simulink model "LLC_Reverse"  (R2024a)
settings: Solver=FixedStepDiscrete  StartTime=0.0  StopTime=0.3  FixedStep=Ts_Power  RelTol=1e-3  EnableMultiTasking=on
values from neighbouring files (symbols this model uses):
  Co = 560e-6    (= 0.00056)    [LLC_Data.m]    (also in LLC_Reverse_Data.m)
  Cr = 140e-9    (= 1.4e-07)    [LLC_Data.m]    (also in LLC_Reverse_Data.m)
  fs_LCC_max = 250e3    (= 250000)    [LLC_Data.m]    (also in LLC_Reverse_Data.m)
  fs_LCC_min = 40e3    (= 40000)    [LLC_Data.m]    (also in LLC_Reverse_Data.m)
  Ki_LLC = 500e3    (= 500000)    [LLC_Data.m]    (also in LLC_Reverse_Data.m)
  Kp_LLC = 5e3    (= 5000)    [LLC_Data.m]    (also in LLC_Reverse_Data.m)
  Lm = 100e-6    (= 0.0001)    [LLC_Data.m]    (also in LLC_Reverse_Data.m)
  Lr = 20e-6    (= 2e-05)    [LLC_Data.m]    (also in LLC_Reverse_Data.m)
  Np = 11    [LLC_Data.m]    (also in LLC_Reverse_Data.m)
  Ns = 10    [LLC_Data.m]    (also in LLC_Reverse_Data.m)
  Ro = Vo_nom^2/Po_nom    (= 19.6363636364)    [LLC_Data.m]    (also in LLC_Reverse_Data.m)
  Ts_Control = 10e-6    (= 1e-05)    [LLC_Data.m]    (also in LLC_Reverse_Data.m)
  Ts_Power = 50e-9    (= 5e-08)    [LLC_Data.m]    (also in LLC_Reverse_Data.m)
  V_o_max = 450    [LLC_Data.m]    (also in LLC_Reverse_Data.m)
  V_o_min = 275    [LLC_Data.m]    (also in LLC_Reverse_Data.m)
undefined symbols (not defined in the file or in its folder): DiscIntNeverNeededParam
libraries: spsMosfetLib x8, spsVoltageMeasurementLib x5, spsSeriesRLCBranchLib x4, spsOnDelayLib x4, spsCurrentMeasurementLib x3, slpidlib x2, spsControlledVoltageSourceLib x1, spsLinearTransformerLib x1, spspowerguiLib x1
settings Model: SimulationMode=accelerator  Creator=LWYohann  LastModifiedBy=LWYohann

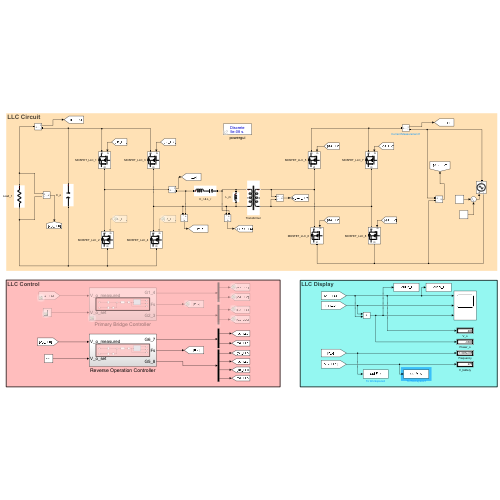
[thumbnail: Simulink's stored preview of the top-level diagram]
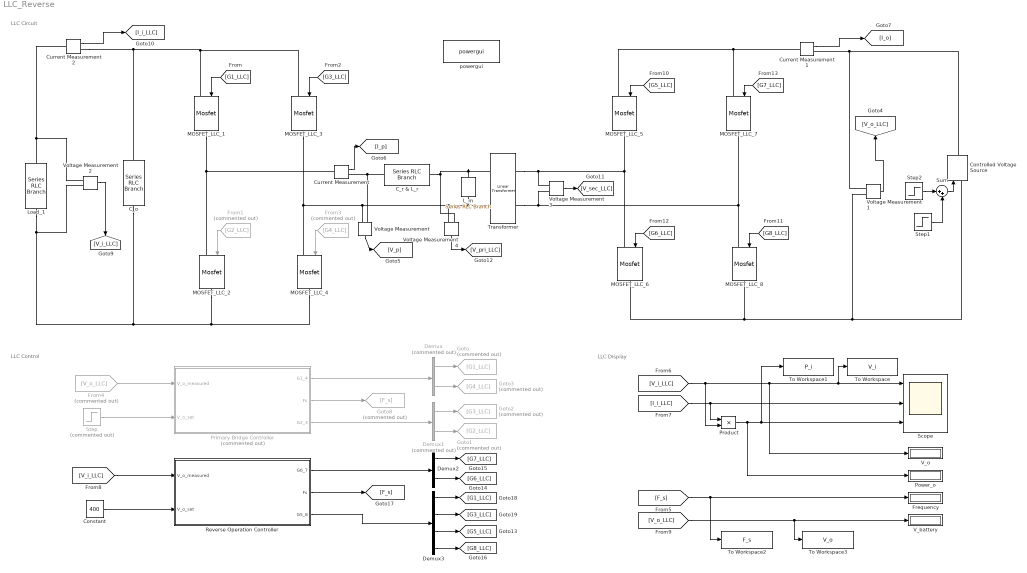
== system LLC_Reverse ==
  note: LLC Display
  note: LLC Control
  note: LLC Circuit
  C_o : spsSeriesRLCBranchLib/Series RLC Branch  LConnTagsString=__new0  RConnTagsString=__new0  BranchType=C  Resistance=1  Inductance=1e-3  SetiL0=off  InitialCurrent=0  Capacitance=Co  Setx0=on  InitialVoltage=400  Measurements=None
  C_r & L_r : spsSeriesRLCBranchLib/Series RLC Branch  LConnTagsString=__new0  RConnTagsString=__new0  BranchType=LC  Resistance=1  Inductance=Lr  SetiL0=off  InitialCurrent=0  Capacitance=Cr  Setx0=off  InitialVoltage=0  Measurements=Branch current
  Constant : Constant  Value=400  SampleTime=Ts_Power
  Controlled Voltage Source : spsControlledVoltageSourceLib/Controlled Voltage Source  Initialize=on  Source_Type=DC  Amplitude=360  Phase=0  Frequency=0  Measurements=None
  Current Measurement : spsCurrentMeasurementLib/Current Measurement  PhasorSimulation=off  OutputType=Complex  PSBequivalent=0
  Current Measurement1 : spsCurrentMeasurementLib/Current Measurement  PhasorSimulation=off  OutputType=Complex  PSBequivalent=0
  Current Measurement2 : spsCurrentMeasurementLib/Current Measurement  PhasorSimulation=off  OutputType=Complex  PSBequivalent=0
  Demux : Demux  Commented=on  Outputs=2
  Demux1 : Demux  Commented=on  Outputs=2
  Demux2 : Demux  Outputs=2
  Demux3 : Demux
  Frequency : Display
  From1 : From  Commented=on  GotoTag=G2_LLC
  From3 : From  Commented=on  GotoTag=G4_LLC
  From4 : From  Commented=on  GotoTag=V_o_LLC
  Goto : Goto  Commented=on  GotoTag=G1_LLC
  Goto1 : Goto  Commented=on  GotoTag=G2_LLC
  Goto2 : Goto  Commented=on  GotoTag=G3_LLC
  Goto3 : Goto  Commented=on  GotoTag=G4_LLC
  Goto8 : Goto  Commented=on  GotoTag=F_s
  L_m : spsSeriesRLCBranchLib/Series RLC Branch  LConnTagsString=__new0  RConnTagsString=__new0  BranchType=L  Resistance=1  Inductance=Lm  SetiL0=off  InitialCurrent=0  Capacitance=Cr  Setx0=off  InitialVoltage=0  Measurements=Branch current
  Load_1 : spsSeriesRLCBranchLib/Series RLC Branch  LConnTagsString=__new0  RConnTagsString=__new0  BranchType=R  Resistance=2*Ro  Inductance=1e-3  SetiL0=off  InitialCurrent=0  Capacitance=Co  Setx0=on  InitialVoltage=375  Measurements=None
  MOSFET_LLC_{1..8} (8 alike) : spsMosfetLib/Mosfet  Ron=Ron_FET  Lon=0  Rd=Ron_Diode  Vfd=Vf  IC=0  Rs=1e6  Cs=inf  Measurements=off
  Power_o : Display
  Primary Bridge Controller : Subsystem  Commented=on
  Product : Product
  Reverse Operation Controller : Subsystem
  Scope : Scope  NumInputPorts=3
  Step : Step  Commented=on  Time=0.1  Before=275  After=360  SampleTime=Ts_Power
  Step1 : Step  Time=0.2  After=-175  SampleTime=Ts_Power
  Step2 : Step  Time=0.1  Before=360  After=450  SampleTime=Ts_Power
  Sum : Sum  Inputs=|++
  To Workspace : ToWorkspace  VariableName=V_i  SaveFormat=Structure With Time  SampleTime=Ts_Power
  To Workspace1 : ToWorkspace  VariableName=P_i  SaveFormat=Structure With Time  SampleTime=Ts_Power
  To Workspace2 : ToWorkspace  VariableName=F_s  SaveFormat=Structure With Time  SampleTime=Ts_Power
  To Workspace3 : ToWorkspace  VariableName=V_o  SaveFormat=Structure With Time  SampleTime=Ts_Power
  Transformer : spsLinearTransformerLib/Linear Transformer  UNITS=SI  NominalPower=[ 6.6e3 100e3 ]  winding1="[Np   1e-2 0]"  winding2="[Ns  1e-2  0 ]"  ThreeWindings=off  winding3=[3.15e+05 0.7938 0.084225]  RmLm=[1e4 0]  Measurements=Magnetization current  DataType=on
  V_battery : Display
  V_o : Display
  Voltage Measurement{,1..4} (5 alike) : spsVoltageMeasurementLib/Voltage Measurement  PhasorSimulation=off  OutputType=Complex  PSBequivalent=0
  powergui : spspowerguiLib/powergui  Priority=1  SimulationMode=Discrete  SampleTime=Ts_Power  frequency=60  Iterations=50  frequencyindice=0  Pbase=100e6  ErrMax=1e-4  UnitsV=kV  UnitsW=MW  buscounter=0  FunctionMessages=off  echomessages=off  EnableUseOfTLC=off  CurrentSourceSwitches=off  DisableSnubberDevices=off  DisableRonSwitches=off  DisableVfSwitches=off  DisplayEquations=off  AutomaticDiscreteSolvers=off  SolverType=Tustin/Backward Euler (TBE)  Interpol=off  ExternalGateDelay=off  methode=off  Ts=100  x0status=blocks  SPID=on  SwTol=0  HookPort=off  NonlinearTolerance=1e-4  nMaxIteration=100  ContinueOnMaxIteration=off  RestoreLinks=warning  ResistiveCurrentMeasurement=off  Frange=[0:2:500]  Ylog=off  Xlog=on  ShowGrid=off  save=off  variable=ZData  structure=0  ZoomFFT=off  StartTime=0.0  cycles=1  DisplayStyle=1  fundamental=60  FreqAxis=off  MaxFrequency=1000  frequencyindicesteady=1  RmsSteady=1  display=off
  wires:
  Demux/1 -> Goto/1
  Demux/2 -> Goto3/1
  Demux1/1 -> Goto2/1
  Demux1/2 -> Goto1/1
  [G1_LLC] -> MOSFET_LLC_1/1
  From1/1 -> MOSFET_LLC_2/1
  [G3_LLC] -> MOSFET_LLC_3/1
  From3/1 -> MOSFET_LLC_4/1
  Voltage Measurement1/1 -> [V_o_LLC]
  Voltage Measurement/1 -> [V_p]
  Current Measurement/1 -> [I_p]
  Current Measurement1/1 -> [I_o]
  [V_i_LLC] -> V_o/1, To Workspace/1, Scope/1, Product/2
  [I_i_LLC] -> Product/1, Scope/2
  Product/1 -> Power_o/1, To Workspace1/1, Scope/3
  [F_s] -> To Workspace2/1, Frequency/1
  Voltage Measurement2/1 -> [V_i_LLC]
  Current Measurement2/1 -> [I_i_LLC]
  Voltage Measurement3/1 -> [V_sec_LLC]
  [G5_LLC] -> MOSFET_LLC_5/1
  [G8_LLC] -> MOSFET_LLC_8/1
  [G6_LLC] -> MOSFET_LLC_6/1
  [G7_LLC] -> MOSFET_LLC_7/1
  Voltage Measurement4/1 -> [V_pri_LLC]
  From4/1 -> Primary Bridge Controller/1(V_o_measured)
  Step/1 -> Primary Bridge Controller/2(V_o_set)
  Primary Bridge Controller/1(G1_4) -> Demux/1
  Primary Bridge Controller/3(G2_3) -> Demux1/1
  Primary Bridge Controller/2(Fs) -> Goto8/1
  [V_i_LLC] -> Reverse Operation Controller/1(V_o_measured)
  Constant/1 -> Reverse Operation Controller/2(V_o_set)
  Reverse Operation Controller/2(Fs) -> [F_s]
  Step2/1 -> Sum/1
  Sum/1 -> Controlled Voltage Source/1
  Step1/1 -> Sum/2
  Reverse Operation Controller/1(G6_7) -> Demux2/1
  Demux2/1 -> [G7_LLC]
  Demux2/2 -> [G6_LLC]
  Reverse Operation Controller/3(G5_8) -> Demux3/1
  Demux3/1 -> [G1_LLC]
  Demux3/2 -> [G3_LLC]
  Demux3/3 -> [G5_LLC]
  Demux3/4 -> [G8_LLC]
  [V_o_LLC] -> To Workspace3/1, V_battery/1
  connections:
  C_r & L_r/RConn1 -- L_m/LConn1 -- Transformer/LConn1 -- Voltage Measurement4/LConn1
  Transformer/LConn2 -- L_m/RConn1 -- Voltage Measurement4/LConn2 -- Voltage Measurement/LConn2 -- MOSFET_LLC_3/RConn1 -- MOSFET_LLC_4/LConn1
  MOSFET_LLC_1/RConn1 -- Current Measurement/LConn1 -- MOSFET_LLC_2/LConn1
  MOSFET_LLC_3/LConn1 -- Current Measurement2/RConn1 -- C_o/LConn1 -- MOSFET_LLC_1/LConn1
  Voltage Measurement2/LConn2 -- Load_1/RConn1 -- C_o/RConn1 -- MOSFET_LLC_4/RConn1 -- MOSFET_LLC_2/RConn1
  Transformer/RConn1 -- Voltage Measurement3/LConn1 -- MOSFET_LLC_6/LConn1 -- MOSFET_LLC_5/RConn1
  Current Measurement1/LConn1 -- MOSFET_LLC_5/LConn1 -- MOSFET_LLC_7/LConn1
  MOSFET_LLC_6/RConn1 -- Voltage Measurement1/LConn2 -- Controlled Voltage Source/LConn1 -- MOSFET_LLC_8/RConn1
  Transformer/RConn2 -- Voltage Measurement3/LConn2 -- MOSFET_LLC_7/RConn1 -- MOSFET_LLC_8/LConn1
  C_r & L_r/LConn1 -- Voltage Measurement/LConn1 -- Current Measurement/RConn1
  Current Measurement2/LConn1 -- Load_1/LConn1 -- Voltage Measurement2/LConn1
  Voltage Measurement1/LConn1 -- Controlled Voltage Source/RConn1 -- Current Measurement1/RConn1

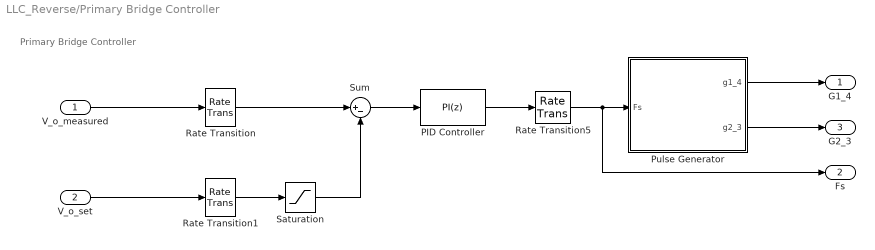
== system LLC_Reverse/Primary Bridge Controller ==
  note: Primary Bridge Controller
  V_o_measured : Inport
  V_o_set : Inport  Port=2
  PID Controller : slpidlib/PID Controller  Controller=PI  Form=Parallel  TimeDomain=Discrete-time  UseExternalTs=off  SampleTime=Ts_Control  IntegratorMethod=Forward Euler  FilterMethod=Forward Euler  ControllerParametersSource=internal  P=Kp_LLC  I=Ki_LLC  UseKiTs=off  D=0  UseExternalDerivativeSource=off  N=100  UseFilter=on  TunerSelectOption=Transfer Function Based (PID Tuner App)  InitialConditionSource=internal  InitialConditionForIntegrator=fr  InitialConditionForFilter=0  DifferentiatorICPrevScaledInput=0  ExternalReset=none  TrackingMode=off  Kt=1  LimitOutput=on  SatLimitsSource=internal  UpperSaturationLimit=fs_LCC_max  LowerSaturationLimit=fs_LCC_min  LinearizeAsGain=on  AntiWindupMode=none  Kb=1  LimitIntegrator=on  UpperIntegratorSaturationLimit=fs_LCC_max  LowerIntegratorSaturationLimit=fs_LCC_min  POutMin=[]  POutMax=[]  IOutMin=[]  IOutMax=[]  DOutMin=[]  DOutMax=[]  NOutMin=[]  NOutMax=[]  SumOutMin=[]  SumOutMax=[]  SaturationOutMin=[]  SaturationOutMax=[]  PParamMin=[]  PParamMax=[]  IParamMin=[]  IParamMax=[]  DParamMin=[]  DParamMax=[]  NParamMin=[]  NParamMax=[]  KbParamMin=[]  KbParamMax=[]  KtParamMin=[]  KtParamMax=[]  KbOutMin=[]  KbOutMax=[]  KtOutMin=[]  KtOutMax=[]  IntegratorOutMin=[]  IntegratorOutMax=[]  FilterOutMin=[]  FilterOutMax=[]  SumI1OutMin=[]  SumI1OutMax=[]  SumI2OutMin=[]  SumI2OutMax=[]  SumI3OutMin=[]  SumI3OutMax=[]  SumI4OutMin=[]  SumI4OutMax=[]  SumDOutMin=[]  SumDOutMax=[]  DifferentiatorOutMin=[]  DifferentiatorOutMax=[]  FilterDiffOutCoefMin=[]  FilterDiffOutCoefMax=[]  ReciprocalOutMin=[]  ReciprocalOutMax=[]  SumDenOutMin=[]  SumDenOutMax=[]  SumNumOutMin=[]  SumNumOutMax=[]  DivideOutMin=[]  DivideOutMax=[]  UdiffTsProdOutMin=[]  UdiffTsProdOutMax=[]  NTsProdOutMin=[]  NTsProdOutMax=[]  UintegralTsProdOutMin=[]  UintegralTsProdOutMax=[]  UngainTsProdOutMin=[]  UngainTsProdOutMax=[]  ClampingZeroOutDataTypeStr=Inherit: Inherit via back propagation  ClampingZeroOutMin=[]  ClampingZeroOutMax=[]  FilterDenConstantOutDataTypeStr=Inherit: Inherit via back propagation  FilterDenConstantOutMin=[]  FilterDenConstantOutMax=[]  PCopyOutDataTypeStr=Inherit: Inherit via back propagation  PCopyOutMin=[]  PCopyOutMax=[]  NCopyOutDataTypeStr=Inherit: Inherit via back propagation  NCopyOutMin=[]  NCopyOutMax=[]  IntegratorContinuousStateAttributes=''  IntegratorStateMustResolveToSignalObject=off  IntegratorRTWStateStorageClass=Auto  FilterContinuousStateAttributes=''  FilterStateMustResolveToSignalObject=off  FilterRTWStateStorageClass=Auto  ParallelPVariant=InternalParameters  IdealPVariant=Disabled  IVariant=InternalParameters  DVariant=Disabled  IntegratorVariant=Discrete  SatVariant=Enabled  AWVariant=Passthrough  PCopyVariant=Disabled  TRVariant=Disabled  FdbkBlocksVariant=Forward  IdealPFdbkVariant=Disabled  SatFdbkVariant=Disabled  DerivativeFilterVariant=Disabled  NVariant=Disabled  NCopyVariant=Disabled_SignalSpec  FilterICVariant=Disabled  IntegratorICVariant=InternalICs  ExternalResetVariant=Disabled  TRSumVariant=Passthrough  SumFdbkVariant=Disabled  SumVariant=Sum_PI  TsampFilterVariant=InternalTs  TsampNgainVariant=Passthrough  TsampIntegralVariant=Disabled_SignalSpec  ExternalSaturationOutDataTypeStr=Inherit: Same as second input  DerivativeSourceVariant=Disabled
  Pulse Generator : Subsystem
  Rate Transition : RateTransition  OutPortSampleTime=Ts_Control
  Rate Transition1 : RateTransition  OutPortSampleTime=Ts_Control
  Rate Transition5 : RateTransition  InitialCondition=fs_LCC_min  OutPortSampleTime=Ts_Power
  Saturation : Saturate  UpperLimit=V_o_max  LowerLimit=V_o_min
  Sum : Sum  Inputs=|+-
  G1_4 : Outport
  Fs : Outport  Port=2
  G2_3 : Outport  Port=3
  wires:
  V_o_measured/1 -> Rate Transition/1
  Pulse Generator/1(g1_4) -> G1_4/1
  Sum/1 -> PID Controller/1
  PID Controller/1 -> Rate Transition5/1
  Rate Transition5/1 -> Fs/1, Pulse Generator/1(Fs)
  Rate Transition/1 -> Sum/1
  V_o_set/1 -> Rate Transition1/1
  Rate Transition1/1 -> Saturation/1
  Saturation/1 -> Sum/2
  Pulse Generator/2(g2_3) -> G2_3/1

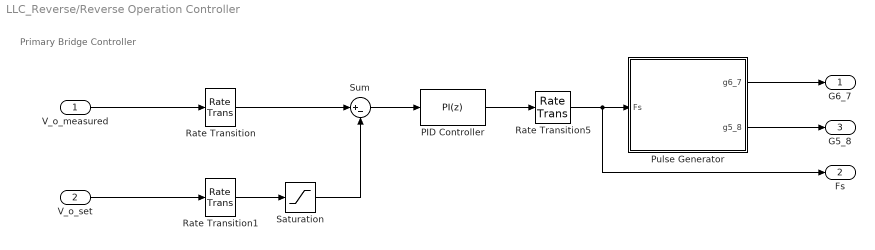
== system LLC_Reverse/Reverse Operation Controller ==
  note: Primary Bridge Controller
  V_o_measured : Inport
  V_o_set : Inport  Port=2
  PID Controller : slpidlib/PID Controller  Controller=PI  Form=Parallel  TimeDomain=Discrete-time  UseExternalTs=off  SampleTime=Ts_Control  IntegratorMethod=Forward Euler  FilterMethod=Forward Euler  ControllerParametersSource=internal  P=Kp_LLC  I=Ki_LLC  UseKiTs=off  D=0  UseExternalDerivativeSource=off  N=100  UseFilter=on  TunerSelectOption=Transfer Function Based (PID Tuner App)  InitialConditionSource=internal  InitialConditionForIntegrator=fr  InitialConditionForFilter=0  DifferentiatorICPrevScaledInput=0  ExternalReset=none  TrackingMode=off  Kt=1  LimitOutput=on  SatLimitsSource=internal  UpperSaturationLimit=fs_LCC_max  LowerSaturationLimit=fs_LCC_min  LinearizeAsGain=on  AntiWindupMode=none  Kb=1  LimitIntegrator=on  UpperIntegratorSaturationLimit=fs_LCC_max  LowerIntegratorSaturationLimit=fs_LCC_min  POutMin=[]  POutMax=[]  IOutMin=[]  IOutMax=[]  DOutMin=[]  DOutMax=[]  NOutMin=[]  NOutMax=[]  SumOutMin=[]  SumOutMax=[]  SaturationOutMin=[]  SaturationOutMax=[]  PParamMin=[]  PParamMax=[]  IParamMin=[]  IParamMax=[]  DParamMin=[]  DParamMax=[]  NParamMin=[]  NParamMax=[]  KbParamMin=[]  KbParamMax=[]  KtParamMin=[]  KtParamMax=[]  KbOutMin=[]  KbOutMax=[]  KtOutMin=[]  KtOutMax=[]  IntegratorOutMin=[]  IntegratorOutMax=[]  FilterOutMin=[]  FilterOutMax=[]  SumI1OutMin=[]  SumI1OutMax=[]  SumI2OutMin=[]  SumI2OutMax=[]  SumI3OutMin=[]  SumI3OutMax=[]  SumI4OutMin=[]  SumI4OutMax=[]  SumDOutMin=[]  SumDOutMax=[]  DifferentiatorOutMin=[]  DifferentiatorOutMax=[]  FilterDiffOutCoefMin=[]  FilterDiffOutCoefMax=[]  ReciprocalOutMin=[]  ReciprocalOutMax=[]  SumDenOutMin=[]  SumDenOutMax=[]  SumNumOutMin=[]  SumNumOutMax=[]  DivideOutMin=[]  DivideOutMax=[]  UdiffTsProdOutMin=[]  UdiffTsProdOutMax=[]  NTsProdOutMin=[]  NTsProdOutMax=[]  UintegralTsProdOutMin=[]  UintegralTsProdOutMax=[]  UngainTsProdOutMin=[]  UngainTsProdOutMax=[]  ClampingZeroOutDataTypeStr=Inherit: Inherit via back propagation  ClampingZeroOutMin=[]  ClampingZeroOutMax=[]  FilterDenConstantOutDataTypeStr=Inherit: Inherit via back propagation  FilterDenConstantOutMin=[]  FilterDenConstantOutMax=[]  PCopyOutDataTypeStr=Inherit: Inherit via back propagation  PCopyOutMin=[]  PCopyOutMax=[]  NCopyOutDataTypeStr=Inherit: Inherit via back propagation  NCopyOutMin=[]  NCopyOutMax=[]  IntegratorContinuousStateAttributes=''  IntegratorStateMustResolveToSignalObject=off  IntegratorRTWStateStorageClass=Auto  FilterContinuousStateAttributes=''  FilterStateMustResolveToSignalObject=off  FilterRTWStateStorageClass=Auto  ParallelPVariant=InternalParameters  IdealPVariant=Disabled  IVariant=InternalParameters  DVariant=Disabled  IntegratorVariant=Discrete  SatVariant=Enabled  AWVariant=Passthrough  PCopyVariant=Disabled  TRVariant=Disabled  FdbkBlocksVariant=Forward  IdealPFdbkVariant=Disabled  SatFdbkVariant=Disabled  DerivativeFilterVariant=Disabled  NVariant=Disabled  NCopyVariant=Disabled_SignalSpec  FilterICVariant=Disabled  IntegratorICVariant=InternalICs  ExternalResetVariant=Disabled  TRSumVariant=Passthrough  SumFdbkVariant=Disabled  SumVariant=Sum_PI  TsampFilterVariant=InternalTs  TsampNgainVariant=Passthrough  TsampIntegralVariant=Disabled_SignalSpec  ExternalSaturationOutDataTypeStr=Inherit: Same as second input  DerivativeSourceVariant=Disabled
  Pulse Generator : Subsystem
  Rate Transition : RateTransition  OutPortSampleTime=Ts_Control
  Rate Transition1 : RateTransition  OutPortSampleTime=Ts_Control
  Rate Transition5 : RateTransition  InitialCondition=fs_LCC_min  OutPortSampleTime=Ts_Power
  Saturation : Saturate  UpperLimit=V_o_max  LowerLimit=V_o_min
  Sum : Sum  Inputs=|+-
  G6_7 : Outport
  Fs : Outport  Port=2
  G5_8 : Outport  Port=3
  wires:
  V_o_measured/1 -> Rate Transition/1
  Pulse Generator/1(g6_7) -> G6_7/1
  Sum/1 -> PID Controller/1
  PID Controller/1 -> Rate Transition5/1
  Rate Transition5/1 -> Fs/1, Pulse Generator/1(Fs)
  Rate Transition/1 -> Sum/1
  V_o_set/1 -> Rate Transition1/1
  Rate Transition1/1 -> Saturation/1
  Saturation/1 -> Sum/2
  Pulse Generator/2(g5_8) -> G5_8/1

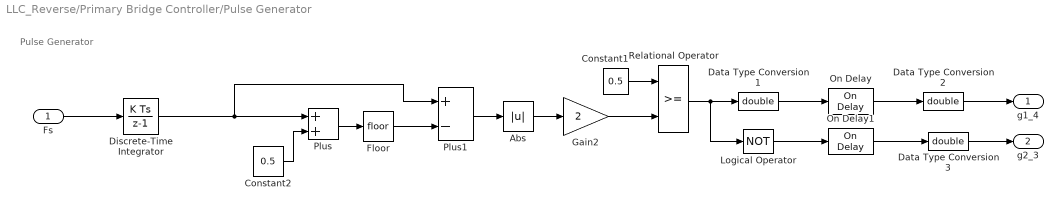
== system LLC_Reverse/Primary Bridge Controller/Pulse Generator ==
  note: Pulse Generator
  Fs : Inport
  Abs : Abs  SaturateOnIntegerOverflow=off
  Constant1 : Constant  Value=0.5
  Constant2 : Constant  Value=0.5
  Data Type Conversion1 : DataTypeConversion  OutDataTypeStr=double  SaturateOnIntegerOverflow=off  RndMeth=Floor
  Data Type Conversion2 : DataTypeConversion  OutDataTypeStr=double  SaturateOnIntegerOverflow=off  RndMeth=Floor
  Data Type Conversion3 : DataTypeConversion  OutDataTypeStr=double  SaturateOnIntegerOverflow=off  RndMeth=Floor
  Discrete-Time Integrator : DiscreteIntegrator  SampleTime=Ts_Power  ICPrevOutput=DiscIntNeverNeededParam  ICPrevScaledInput=DiscIntNeverNeededParam
  Floor : Rounding
  Gain2 : Gain  Gain=2  SaturateOnIntegerOverflow=on  OutDataTypeStr=Inherit: Same as input  ParamDataTypeStr=Inherit: Same as input
  Logical Operator : Logic  Operator=NOT  AllPortsSameDT=off  OutDataTypeStr=float('double')
  On Delay : spsOnDelayLib/On Delay  DelayType=On delay  delay=DT_LLC  ic=0  Ts=Ts_Power
  On Delay1 : spsOnDelayLib/On Delay  DelayType=On delay  delay=DT_LLC  ic=0  Ts=Ts_Power
  Plus : Sum
  Plus1 : Sum  Inputs=+-
  Relational Operator : RelationalOperator  OutDataTypeStr=boolean  InputSameDT=off
  g1_4 : Outport  VectorParamsAs1DForOutWhenUnconnected=off
  g2_3 : Outport  Port=2  VectorParamsAs1DForOutWhenUnconnected=off
  wires:
  On Delay1/1 -> Data Type Conversion3/1
  On Delay/1 -> Data Type Conversion2/1
  Data Type Conversion1/1 -> On Delay/1
  Logical Operator/1 -> On Delay1/1
  Gain2/1 -> Relational Operator/2
  Relational Operator/1 -> Logical Operator/1, Data Type Conversion1/1
  Constant1/1 -> Relational Operator/1
  Data Type Conversion2/1 -> g1_4/1
  Data Type Conversion3/1 -> g2_3/1
  Plus/1 -> Floor/1
  Discrete-Time Integrator/1 -> Plus1/1, Plus/1
  Abs/1 -> Gain2/1
  Floor/1 -> Plus1/2
  Plus1/1 -> Abs/1
  Fs/1 -> Discrete-Time Integrator/1
  Constant2/1 -> Plus/2

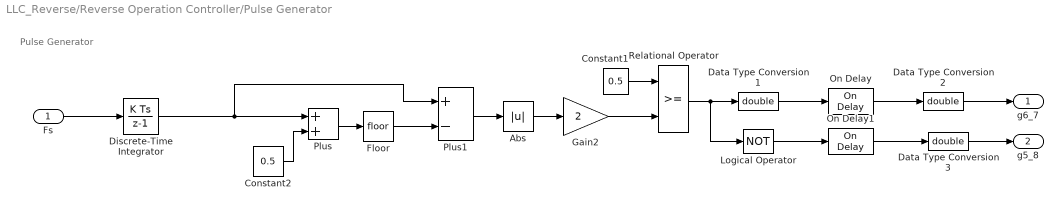
== system LLC_Reverse/Reverse Operation Controller/Pulse Generator ==
  note: Pulse Generator
  Fs : Inport
  Abs : Abs  SaturateOnIntegerOverflow=off
  Constant1 : Constant  Value=0.5
  Constant2 : Constant  Value=0.5
  Data Type Conversion1 : DataTypeConversion  OutDataTypeStr=double  SaturateOnIntegerOverflow=off  RndMeth=Floor
  Data Type Conversion2 : DataTypeConversion  OutDataTypeStr=double  SaturateOnIntegerOverflow=off  RndMeth=Floor
  Data Type Conversion3 : DataTypeConversion  OutDataTypeStr=double  SaturateOnIntegerOverflow=off  RndMeth=Floor
  Discrete-Time Integrator : DiscreteIntegrator  SampleTime=Ts_Power  ICPrevOutput=DiscIntNeverNeededParam  ICPrevScaledInput=DiscIntNeverNeededParam
  Floor : Rounding
  Gain2 : Gain  Gain=2  SaturateOnIntegerOverflow=on  OutDataTypeStr=Inherit: Same as input  ParamDataTypeStr=Inherit: Same as input
  Logical Operator : Logic  Operator=NOT  AllPortsSameDT=off  OutDataTypeStr=float('double')
  On Delay : spsOnDelayLib/On Delay  DelayType=On delay  delay=DT_LLC  ic=0  Ts=Ts_Power
  On Delay1 : spsOnDelayLib/On Delay  DelayType=On delay  delay=DT_LLC  ic=0  Ts=Ts_Power
  Plus : Sum
  Plus1 : Sum  Inputs=+-
  Relational Operator : RelationalOperator  OutDataTypeStr=boolean  InputSameDT=off
  g6_7 : Outport  VectorParamsAs1DForOutWhenUnconnected=off
  g5_8 : Outport  Port=2  VectorParamsAs1DForOutWhenUnconnected=off
  wires:
  On Delay1/1 -> Data Type Conversion3/1
  On Delay/1 -> Data Type Conversion2/1
  Data Type Conversion1/1 -> On Delay/1
  Logical Operator/1 -> On Delay1/1
  Gain2/1 -> Relational Operator/2
  Relational Operator/1 -> Logical Operator/1, Data Type Conversion1/1
  Constant1/1 -> Relational Operator/1
  Data Type Conversion2/1 -> g6_7/1
  Data Type Conversion3/1 -> g5_8/1
  Plus/1 -> Floor/1
  Discrete-Time Integrator/1 -> Plus1/1, Plus/1
  Abs/1 -> Gain2/1
  Floor/1 -> Plus1/2
  Plus1/1 -> Abs/1
  Fs/1 -> Discrete-Time Integrator/1
  Constant2/1 -> Plus/2
